simulink model "TST_InjCrv_MI1"  (R2016b)
settings: Solver=FixedStepDiscrete  StartTime=0.0  StopTime=simTime  FixedStep=sampleTime  RelTol=1e-3
values from neighbouring files (symbols this model uses):
  testCase = 1    [initTST_InjCrv_MI1_001.m]    (also in initTST_InjCrv_MI1_002.m = 2; initTST_InjCrv_MI1_003.m = 3; initTST_InjCrv_MI1_004.m = 4; initTST_InjCrv_MI1_005.m = 5)
libraries: simulink x26, UnitTest_Lib x20
settings Model: Creator=zhengjinyan  LastModifiedBy=zhengjinyan
settings DebuggingCC: SignalRangeChecking=error

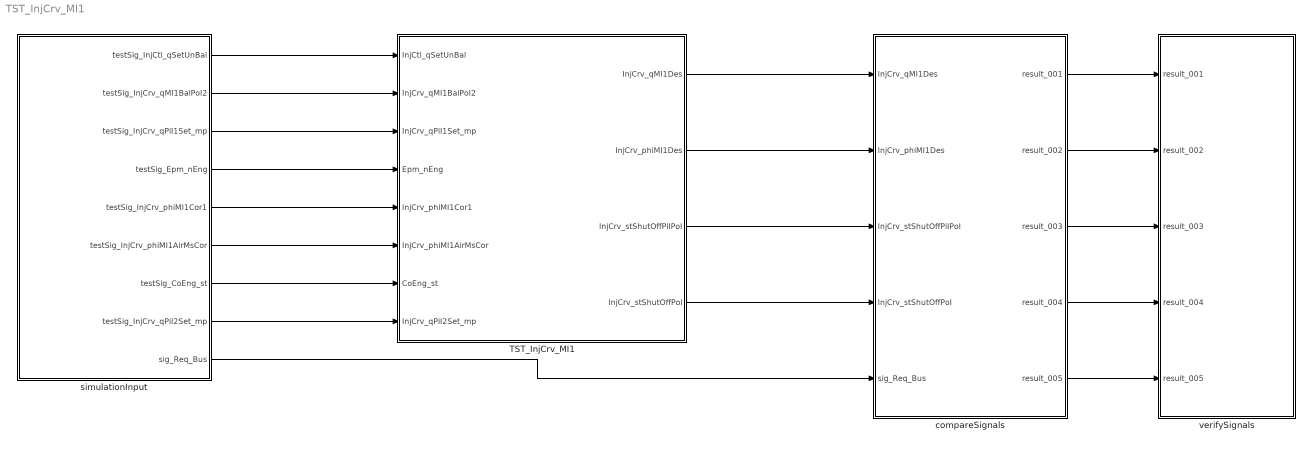
== system TST_InjCrv_MI1 ==
  TST_InjCrv_MI1 : Subsystem
  compareSignals : Subsystem
  simulationInput : Subsystem
  verifySignals : Subsystem
  wires:
  simulationInput/1(testSig_InjCtl_qSetUnBal) -> TST_InjCrv_MI1/1(InjCtl_qSetUnBal)
  simulationInput/2(testSig_InjCrv_qMI1BalPoI2) -> TST_InjCrv_MI1/2(InjCrv_qMI1BalPoI2)
  simulationInput/3(testSig_InjCrv_qPiI1Set_mp) -> TST_InjCrv_MI1/3(InjCrv_qPiI1Set_mp)
  simulationInput/4(testSig_Epm_nEng) -> TST_InjCrv_MI1/4(Epm_nEng)
  simulationInput/5(testSig_InjCrv_phiMI1Cor1) -> TST_InjCrv_MI1/5(InjCrv_phiMI1Cor1)
  simulationInput/6(testSig_InjCrv_phiMI1AirMsCor) -> TST_InjCrv_MI1/6(InjCrv_phiMI1AirMsCor)
  simulationInput/7(testSig_CoEng_st) -> TST_InjCrv_MI1/7(CoEng_st)
  simulationInput/8(testSig_InjCrv_qPiI2Set_mp) -> TST_InjCrv_MI1/8(InjCrv_qPiI2Set_mp)
  TST_InjCrv_MI1/1(InjCrv_qMI1Des) -> compareSignals/1(InjCrv_qMI1Des)
  TST_InjCrv_MI1/2(InjCrv_phiMI1Des) -> compareSignals/2(InjCrv_phiMI1Des)
  TST_InjCrv_MI1/3(InjCrv_stShutOffPiIPoI) -> compareSignals/3(InjCrv_stShutOffPiIPoI)
  TST_InjCrv_MI1/4(InjCrv_stShutOffPoI) -> compareSignals/4(InjCrv_stShutOffPoI)
  simulationInput/9(sig_Req_Bus) -> compareSignals/5(sig_Req_Bus)
  compareSignals/1(result_001) -> verifySignals/1(result_001)
  compareSignals/2(result_002) -> verifySignals/2(result_002)
  compareSignals/3(result_003) -> verifySignals/3(result_003)
  compareSignals/4(result_004) -> verifySignals/4(result_004)
  compareSignals/5(result_005) -> verifySignals/5(result_005)

== system TST_InjCrv_MI1/TST_InjCrv_MI1 ==
  InjCtl_qSetUnBal : Inport
  InjCrv_qMI1BalPoI2 : Inport  Port=2
  InjCrv_qPiI1Set_mp : Inport  Port=3
  Epm_nEng : Inport  Port=4
  InjCrv_phiMI1Cor1 : Inport  Port=5
  InjCrv_phiMI1AirMsCor : Inport  Port=6
  CoEng_st : Inport  Port=7
  InjCrv_qPiI2Set_mp : Inport  Port=8
  Function_Call : simulink/Ports & Subsystems/Function-Call Generator  sample_time=sampleTime  numberOfIterations=1
  InjCrv_MI1 : ModelReference  ModelNameDialog=InjCrv_MI1  SimulationMode=Normal  ModelReferenceVersion=1.46  TriggerPortName=function  TriggerPortTriggerType=function-call  TriggerPortStatesWhenEnabling=held
  InjCrv_qMI1Des : Outport
  InjCrv_phiMI1Des : Outport  Port=2
  InjCrv_stShutOffPiIPoI : Outport  Port=3
  InjCrv_stShutOffPoI : Outport  Port=4
  wires:
  Function_Call/1 -> InjCrv_MI1/Trigger
  InjCtl_qSetUnBal/1 -> InjCrv_MI1/1
  InjCrv_qMI1BalPoI2/1 -> InjCrv_MI1/2
  InjCrv_qPiI1Set_mp/1 -> InjCrv_MI1/3
  Epm_nEng/1 -> InjCrv_MI1/4
  InjCrv_phiMI1Cor1/1 -> InjCrv_MI1/5
  InjCrv_phiMI1AirMsCor/1 -> InjCrv_MI1/6
  CoEng_st/1 -> InjCrv_MI1/7
  InjCrv_qPiI2Set_mp/1 -> InjCrv_MI1/8
  InjCrv_MI1/1 -> InjCrv_qMI1Des/1
  InjCrv_MI1/2 -> InjCrv_phiMI1Des/1
  InjCrv_MI1/3 -> InjCrv_stShutOffPiIPoI/1
  InjCrv_MI1/4 -> InjCrv_stShutOffPoI/1

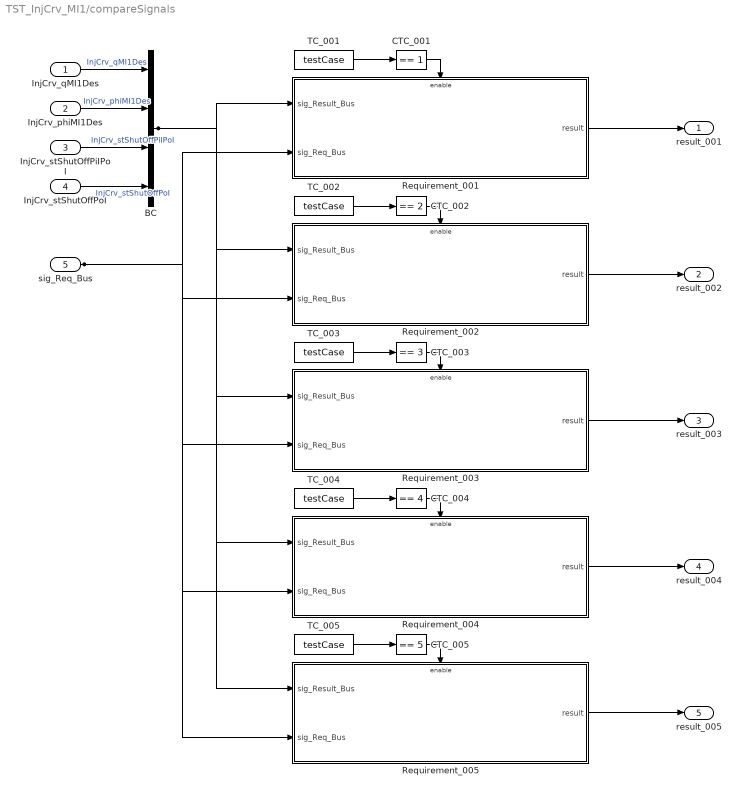
== system TST_InjCrv_MI1/compareSignals ==
  InjCrv_qMI1Des : Inport
  InjCrv_phiMI1Des : Inport  Port=2
  InjCrv_stShutOffPiIPoI : Inport  Port=3
  InjCrv_stShutOffPoI : Inport  Port=4
  sig_Req_Bus : Inport  Port=5
  BC : BusCreator  Inputs=4
  CTC_001 : simulink/Logic and Bit Operations/Compare To Constant  relop===  const=1  OutDataTypeStr=boolean
  CTC_002 : simulink/Logic and Bit Operations/Compare To Constant  relop===  const=2  OutDataTypeStr=boolean
  CTC_003 : simulink/Logic and Bit Operations/Compare To Constant  relop===  const=3  OutDataTypeStr=boolean
  CTC_004 : simulink/Logic and Bit Operations/Compare To Constant  relop===  const=4  OutDataTypeStr=boolean
  CTC_005 : simulink/Logic and Bit Operations/Compare To Constant  relop===  const=5  OutDataTypeStr=boolean
  Requirement_001 : Subsystem
  Requirement_002 : Subsystem
  Requirement_003 : Subsystem
  Requirement_004 : Subsystem
  Requirement_005 : Subsystem
  TC_001 : Constant  Value=testCase
  TC_002 : Constant  Value=testCase
  TC_003 : Constant  Value=testCase
  TC_004 : Constant  Value=testCase
  TC_005 : Constant  Value=testCase
  result_001 : Outport
  result_002 : Outport  Port=2
  result_003 : Outport  Port=3
  result_004 : Outport  Port=4
  result_005 : Outport  Port=5
  wires:
  InjCrv_qMI1Des/1 -> BC/1  "InjCrv_qMI1Des"
  InjCrv_phiMI1Des/1 -> BC/2  "InjCrv_phiMI1Des"
  InjCrv_stShutOffPiIPoI/1 -> BC/3  "InjCrv_stShutOffPiIPoI"
  InjCrv_stShutOffPoI/1 -> BC/4  "InjCrv_stShutOffPoI"
  TC_001/1 -> CTC_001/1
  CTC_001/1 -> Requirement_001/Enable
  sig_Req_Bus/1 -> Requirement_001/2(sig_Req_Bus), Requirement_002/2(sig_Req_Bus), Requirement_003/2(sig_Req_Bus), Requirement_004/2(sig_Req_Bus), Requirement_005/2(sig_Req_Bus)
  BC/1 -> Requirement_001/1(sig_Result_Bus), Requirement_002/1(sig_Result_Bus), Requirement_003/1(sig_Result_Bus), Requirement_004/1(sig_Result_Bus), Requirement_005/1(sig_Result_Bus)
  Requirement_001/1(result) -> result_001/1
  TC_002/1 -> CTC_002/1
  CTC_002/1 -> Requirement_002/Enable
  Requirement_002/1(result) -> result_002/1
  TC_003/1 -> CTC_003/1
  CTC_003/1 -> Requirement_003/Enable
  Requirement_003/1(result) -> result_003/1
  TC_004/1 -> CTC_004/1
  CTC_004/1 -> Requirement_004/Enable
  Requirement_004/1(result) -> result_004/1
  TC_005/1 -> CTC_005/1
  CTC_005/1 -> Requirement_005/Enable
  Requirement_005/1(result) -> result_005/1

== system TST_InjCrv_MI1/simulationInput ==
  BS : BusSelector  OutputSignals=testSig_InjCtl_qSetUnBal,testSig_InjCrv_qMI1BalPoI2,testSig_InjCrv_qPiI1Set_mp,testSig_Epm_nEng,testSig_InjCrv_phiMI1Cor1,testSig_InjCrv_phiMI1AirMsCor,testSig_CoEng_st,testSig_InjCrv_qPiI2Set_mp
  MPSw : MultiPortSwitch  Inputs=5  SaturateOnIntegerOverflow=on  InputSameDT=on
  TestCase : Constant  Value=testCase
  testSignals_R001 : Subsystem
  testSignals_R002 : Subsystem
  testSignals_R003 : Subsystem
  testSignals_R004 : Subsystem
  testSignals_R005 : Subsystem
  testSig_InjCtl_qSetUnBal : Outport
  testSig_InjCrv_qMI1BalPoI2 : Outport  Port=2
  testSig_InjCrv_qPiI1Set_mp : Outport  Port=3
  testSig_Epm_nEng : Outport  Port=4
  testSig_InjCrv_phiMI1Cor1 : Outport  Port=5
  testSig_InjCrv_phiMI1AirMsCor : Outport  Port=6
  testSig_CoEng_st : Outport  Port=7
  testSig_InjCrv_qPiI2Set_mp : Outport  Port=8
  sig_Req_Bus : Outport  Port=9
  wires:
  BS/1 -> testSig_InjCtl_qSetUnBal/1  "<testSig_InjCtl_qSetUnBal>"
  BS/2 -> testSig_InjCrv_qMI1BalPoI2/1  "<testSig_InjCrv_qMI1BalPoI2>"
  BS/3 -> testSig_InjCrv_qPiI1Set_mp/1  "<testSig_InjCrv_qPiI1Set_mp>"
  BS/4 -> testSig_Epm_nEng/1  "<testSig_Epm_nEng>"
  BS/5 -> testSig_InjCrv_phiMI1Cor1/1  "<testSig_InjCrv_phiMI1Cor1>"
  BS/6 -> testSig_InjCrv_phiMI1AirMsCor/1  "<testSig_InjCrv_phiMI1AirMsCor>"
  BS/7 -> testSig_CoEng_st/1  "<testSig_CoEng_st>"
  BS/8 -> testSig_InjCrv_qPiI2Set_mp/1  "<testSig_InjCrv_qPiI2Set_mp>"
  MPSw/1 -> BS/1, sig_Req_Bus/1
  TestCase/1 -> MPSw/1
  testSignals_R001/1(testSignals) -> MPSw/2
  testSignals_R002/1(testSignals) -> MPSw/3
  testSignals_R003/1(testSignals) -> MPSw/4
  testSignals_R004/1(testSignals) -> MPSw/5
  testSignals_R005/1(testSignals) -> MPSw/6

== system TST_InjCrv_MI1/verifySignals ==
  result_001 : Inport
  result_002 : Inport  Port=2
  result_003 : Inport  Port=3
  result_004 : Inport  Port=4
  result_005 : Inport  Port=5
  Assertion_001 : Assertion  Enabled=off
  Assertion_002 : Assertion  Enabled=off
  Assertion_003 : Assertion  Enabled=off
  Assertion_004 : Assertion  Enabled=off
  Assertion_005 : Assertion  Enabled=off
  wires:
  result_001/1 -> Assertion_001/1
  result_002/1 -> Assertion_002/1
  result_003/1 -> Assertion_003/1
  result_004/1 -> Assertion_004/1
  result_005/1 -> Assertion_005/1

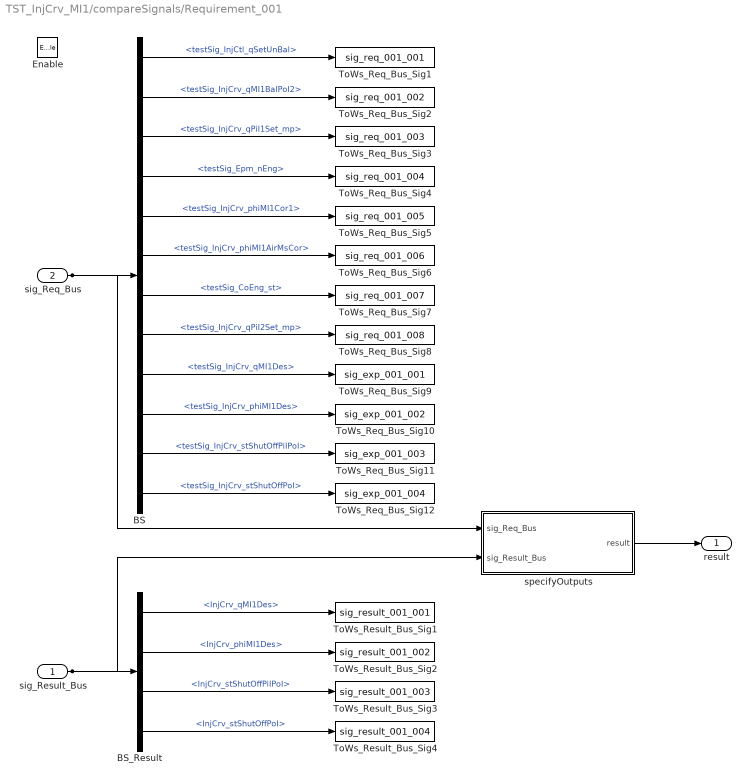
== system TST_InjCrv_MI1/compareSignals/Requirement_001 ==
  sig_Result_Bus : Inport
  sig_Req_Bus : Inport  Port=2
  Enable : EnablePort
  BS : BusSelector  OutputSignals=testSig_InjCtl_qSetUnBal,testSig_InjCrv_qMI1BalPoI2,testSig_InjCrv_qPiI1Set_mp,testSig_Epm_nEng,testSig_InjCrv_phiMI1Cor1,testSig_InjCrv_phiMI1AirMsCor,testSig_CoEng_st,testSig_InjCrv_qPiI2Set_mp,testSig_InjCrv_qMI1Des,testSig_InjCrv_phiMI1Des,testSig_InjCrv_stShutOffPiIPoI,testSig_InjCrv_stShutOffPoI
  BS_Result : BusSelector  OutputSignals=InjCrv_qMI1Des,InjCrv_phiMI1Des,InjCrv_stShutOffPiIPoI,InjCrv_stShutOffPoI
  ToWs_Req_Bus_Sig1 : ToWorkspace  VariableName=sig_req_001_001  SaveFormat=Structure With Time
  ToWs_Req_Bus_Sig10 : ToWorkspace  VariableName=sig_exp_001_002  SaveFormat=Structure With Time
  ToWs_Req_Bus_Sig11 : ToWorkspace  VariableName=sig_exp_001_003  SaveFormat=Structure With Time
  ToWs_Req_Bus_Sig12 : ToWorkspace  VariableName=sig_exp_001_004  SaveFormat=Structure With Time
  ToWs_Req_Bus_Sig2 : ToWorkspace  VariableName=sig_req_001_002  SaveFormat=Structure With Time
  ToWs_Req_Bus_Sig3 : ToWorkspace  VariableName=sig_req_001_003  SaveFormat=Structure With Time
  ToWs_Req_Bus_Sig4 : ToWorkspace  VariableName=sig_req_001_004  SaveFormat=Structure With Time
  ToWs_Req_Bus_Sig5 : ToWorkspace  VariableName=sig_req_001_005  SaveFormat=Structure With Time
  ToWs_Req_Bus_Sig6 : ToWorkspace  VariableName=sig_req_001_006  SaveFormat=Structure With Time
  ToWs_Req_Bus_Sig7 : ToWorkspace  VariableName=sig_req_001_007  SaveFormat=Structure With Time
  ToWs_Req_Bus_Sig8 : ToWorkspace  VariableName=sig_req_001_008  SaveFormat=Structure With Time
  ToWs_Req_Bus_Sig9 : ToWorkspace  VariableName=sig_exp_001_001  SaveFormat=Structure With Time
  ToWs_Result_Bus_Sig1 : ToWorkspace  VariableName=sig_result_001_001  SaveFormat=Structure With Time
  ToWs_Result_Bus_Sig2 : ToWorkspace  VariableName=sig_result_001_002  SaveFormat=Structure With Time
  ToWs_Result_Bus_Sig3 : ToWorkspace  VariableName=sig_result_001_003  SaveFormat=Structure With Time
  ToWs_Result_Bus_Sig4 : ToWorkspace  VariableName=sig_result_001_004  SaveFormat=Structure With Time
  specifyOutputs : Subsystem
  result : Outport
  wires:
  sig_Req_Bus/1 -> BS/1, specifyOutputs/1(sig_Req_Bus)
  BS/1 -> ToWs_Req_Bus_Sig1/1  "<testSig_InjCtl_qSetUnBal>"
  BS/2 -> ToWs_Req_Bus_Sig2/1  "<testSig_InjCrv_qMI1BalPoI2>"
  BS/3 -> ToWs_Req_Bus_Sig3/1  "<testSig_InjCrv_qPiI1Set_mp>"
  BS/4 -> ToWs_Req_Bus_Sig4/1  "<testSig_Epm_nEng>"
  BS/5 -> ToWs_Req_Bus_Sig5/1  "<testSig_InjCrv_phiMI1Cor1>"
  BS/6 -> ToWs_Req_Bus_Sig6/1  "<testSig_InjCrv_phiMI1AirMsCor>"
  BS/7 -> ToWs_Req_Bus_Sig7/1  "<testSig_CoEng_st>"
  BS/8 -> ToWs_Req_Bus_Sig8/1  "<testSig_InjCrv_qPiI2Set_mp>"
  BS/9 -> ToWs_Req_Bus_Sig9/1  "<testSig_InjCrv_qMI1Des>"
  BS/10 -> ToWs_Req_Bus_Sig10/1  "<testSig_InjCrv_phiMI1Des>"
  BS/11 -> ToWs_Req_Bus_Sig11/1  "<testSig_InjCrv_stShutOffPiIPoI>"
  BS/12 -> ToWs_Req_Bus_Sig12/1  "<testSig_InjCrv_stShutOffPoI>"
  sig_Result_Bus/1 -> BS_Result/1, specifyOutputs/2(sig_Result_Bus)
  BS_Result/1 -> ToWs_Result_Bus_Sig1/1  "<InjCrv_qMI1Des>"
  BS_Result/2 -> ToWs_Result_Bus_Sig2/1  "<InjCrv_phiMI1Des>"
  BS_Result/3 -> ToWs_Result_Bus_Sig3/1  "<InjCrv_stShutOffPiIPoI>"
  BS_Result/4 -> ToWs_Result_Bus_Sig4/1  "<InjCrv_stShutOffPoI>"
  specifyOutputs/1(result) -> result/1

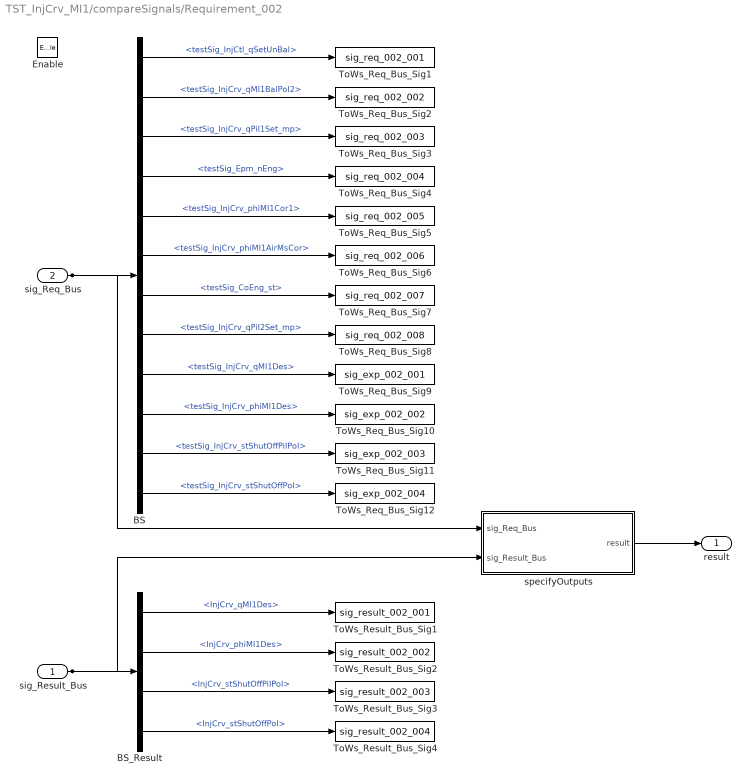
== system TST_InjCrv_MI1/compareSignals/Requirement_002 ==
  sig_Result_Bus : Inport
  sig_Req_Bus : Inport  Port=2
  Enable : EnablePort
  BS : BusSelector  OutputSignals=testSig_InjCtl_qSetUnBal,testSig_InjCrv_qMI1BalPoI2,testSig_InjCrv_qPiI1Set_mp,testSig_Epm_nEng,testSig_InjCrv_phiMI1Cor1,testSig_InjCrv_phiMI1AirMsCor,testSig_CoEng_st,testSig_InjCrv_qPiI2Set_mp,testSig_InjCrv_qMI1Des,testSig_InjCrv_phiMI1Des,testSig_InjCrv_stShutOffPiIPoI,testSig_InjCrv_stShutOffPoI
  BS_Result : BusSelector  OutputSignals=InjCrv_qMI1Des,InjCrv_phiMI1Des,InjCrv_stShutOffPiIPoI,InjCrv_stShutOffPoI
  ToWs_Req_Bus_Sig1 : ToWorkspace  VariableName=sig_req_002_001  SaveFormat=Structure With Time
  ToWs_Req_Bus_Sig10 : ToWorkspace  VariableName=sig_exp_002_002  SaveFormat=Structure With Time
  ToWs_Req_Bus_Sig11 : ToWorkspace  VariableName=sig_exp_002_003  SaveFormat=Structure With Time
  ToWs_Req_Bus_Sig12 : ToWorkspace  VariableName=sig_exp_002_004  SaveFormat=Structure With Time
  ToWs_Req_Bus_Sig2 : ToWorkspace  VariableName=sig_req_002_002  SaveFormat=Structure With Time
  ToWs_Req_Bus_Sig3 : ToWorkspace  VariableName=sig_req_002_003  SaveFormat=Structure With Time
  ToWs_Req_Bus_Sig4 : ToWorkspace  VariableName=sig_req_002_004  SaveFormat=Structure With Time
  ToWs_Req_Bus_Sig5 : ToWorkspace  VariableName=sig_req_002_005  SaveFormat=Structure With Time
  ToWs_Req_Bus_Sig6 : ToWorkspace  VariableName=sig_req_002_006  SaveFormat=Structure With Time
  ToWs_Req_Bus_Sig7 : ToWorkspace  VariableName=sig_req_002_007  SaveFormat=Structure With Time
  ToWs_Req_Bus_Sig8 : ToWorkspace  VariableName=sig_req_002_008  SaveFormat=Structure With Time
  ToWs_Req_Bus_Sig9 : ToWorkspace  VariableName=sig_exp_002_001  SaveFormat=Structure With Time
  ToWs_Result_Bus_Sig1 : ToWorkspace  VariableName=sig_result_002_001  SaveFormat=Structure With Time
  ToWs_Result_Bus_Sig2 : ToWorkspace  VariableName=sig_result_002_002  SaveFormat=Structure With Time
  ToWs_Result_Bus_Sig3 : ToWorkspace  VariableName=sig_result_002_003  SaveFormat=Structure With Time
  ToWs_Result_Bus_Sig4 : ToWorkspace  VariableName=sig_result_002_004  SaveFormat=Structure With Time
  specifyOutputs : Subsystem
  result : Outport
  wires:
  sig_Req_Bus/1 -> BS/1, specifyOutputs/1(sig_Req_Bus)
  BS/1 -> ToWs_Req_Bus_Sig1/1  "<testSig_InjCtl_qSetUnBal>"
  BS/2 -> ToWs_Req_Bus_Sig2/1  "<testSig_InjCrv_qMI1BalPoI2>"
  BS/3 -> ToWs_Req_Bus_Sig3/1  "<testSig_InjCrv_qPiI1Set_mp>"
  BS/4 -> ToWs_Req_Bus_Sig4/1  "<testSig_Epm_nEng>"
  BS/5 -> ToWs_Req_Bus_Sig5/1  "<testSig_InjCrv_phiMI1Cor1>"
  BS/6 -> ToWs_Req_Bus_Sig6/1  "<testSig_InjCrv_phiMI1AirMsCor>"
  BS/7 -> ToWs_Req_Bus_Sig7/1  "<testSig_CoEng_st>"
  BS/8 -> ToWs_Req_Bus_Sig8/1  "<testSig_InjCrv_qPiI2Set_mp>"
  BS/9 -> ToWs_Req_Bus_Sig9/1  "<testSig_InjCrv_qMI1Des>"
  BS/10 -> ToWs_Req_Bus_Sig10/1  "<testSig_InjCrv_phiMI1Des>"
  BS/11 -> ToWs_Req_Bus_Sig11/1  "<testSig_InjCrv_stShutOffPiIPoI>"
  BS/12 -> ToWs_Req_Bus_Sig12/1  "<testSig_InjCrv_stShutOffPoI>"
  sig_Result_Bus/1 -> BS_Result/1, specifyOutputs/2(sig_Result_Bus)
  BS_Result/1 -> ToWs_Result_Bus_Sig1/1  "<InjCrv_qMI1Des>"
  BS_Result/2 -> ToWs_Result_Bus_Sig2/1  "<InjCrv_phiMI1Des>"
  BS_Result/3 -> ToWs_Result_Bus_Sig3/1  "<InjCrv_stShutOffPiIPoI>"
  BS_Result/4 -> ToWs_Result_Bus_Sig4/1  "<InjCrv_stShutOffPoI>"
  specifyOutputs/1(result) -> result/1

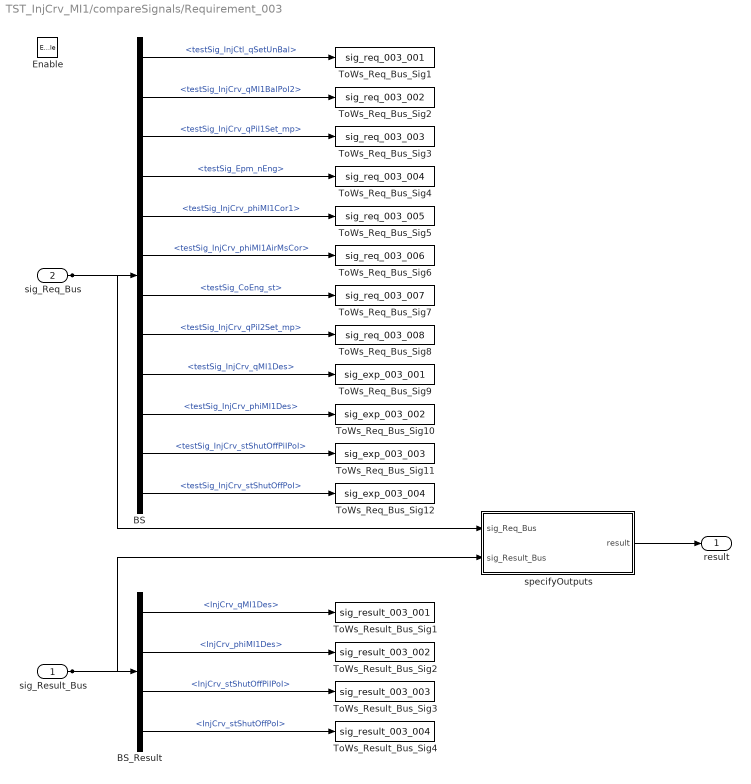
== system TST_InjCrv_MI1/compareSignals/Requirement_003 ==
  sig_Result_Bus : Inport
  sig_Req_Bus : Inport  Port=2
  Enable : EnablePort
  BS : BusSelector  OutputSignals=testSig_InjCtl_qSetUnBal,testSig_InjCrv_qMI1BalPoI2,testSig_InjCrv_qPiI1Set_mp,testSig_Epm_nEng,testSig_InjCrv_phiMI1Cor1,testSig_InjCrv_phiMI1AirMsCor,testSig_CoEng_st,testSig_InjCrv_qPiI2Set_mp,testSig_InjCrv_qMI1Des,testSig_InjCrv_phiMI1Des,testSig_InjCrv_stShutOffPiIPoI,testSig_InjCrv_stShutOffPoI
  BS_Result : BusSelector  OutputSignals=InjCrv_qMI1Des,InjCrv_phiMI1Des,InjCrv_stShutOffPiIPoI,InjCrv_stShutOffPoI
  ToWs_Req_Bus_Sig1 : ToWorkspace  VariableName=sig_req_003_001  SaveFormat=Structure With Time
  ToWs_Req_Bus_Sig10 : ToWorkspace  VariableName=sig_exp_003_002  SaveFormat=Structure With Time
  ToWs_Req_Bus_Sig11 : ToWorkspace  VariableName=sig_exp_003_003  SaveFormat=Structure With Time
  ToWs_Req_Bus_Sig12 : ToWorkspace  VariableName=sig_exp_003_004  SaveFormat=Structure With Time
  ToWs_Req_Bus_Sig2 : ToWorkspace  VariableName=sig_req_003_002  SaveFormat=Structure With Time
  ToWs_Req_Bus_Sig3 : ToWorkspace  VariableName=sig_req_003_003  SaveFormat=Structure With Time
  ToWs_Req_Bus_Sig4 : ToWorkspace  VariableName=sig_req_003_004  SaveFormat=Structure With Time
  ToWs_Req_Bus_Sig5 : ToWorkspace  VariableName=sig_req_003_005  SaveFormat=Structure With Time
  ToWs_Req_Bus_Sig6 : ToWorkspace  VariableName=sig_req_003_006  SaveFormat=Structure With Time
  ToWs_Req_Bus_Sig7 : ToWorkspace  VariableName=sig_req_003_007  SaveFormat=Structure With Time
  ToWs_Req_Bus_Sig8 : ToWorkspace  VariableName=sig_req_003_008  SaveFormat=Structure With Time
  ToWs_Req_Bus_Sig9 : ToWorkspace  VariableName=sig_exp_003_001  SaveFormat=Structure With Time
  ToWs_Result_Bus_Sig1 : ToWorkspace  VariableName=sig_result_003_001  SaveFormat=Structure With Time
  ToWs_Result_Bus_Sig2 : ToWorkspace  VariableName=sig_result_003_002  SaveFormat=Structure With Time
  ToWs_Result_Bus_Sig3 : ToWorkspace  VariableName=sig_result_003_003  SaveFormat=Structure With Time
  ToWs_Result_Bus_Sig4 : ToWorkspace  VariableName=sig_result_003_004  SaveFormat=Structure With Time
  specifyOutputs : Subsystem
  result : Outport
  wires:
  sig_Req_Bus/1 -> BS/1, specifyOutputs/1(sig_Req_Bus)
  BS/1 -> ToWs_Req_Bus_Sig1/1  "<testSig_InjCtl_qSetUnBal>"
  BS/2 -> ToWs_Req_Bus_Sig2/1  "<testSig_InjCrv_qMI1BalPoI2>"
  BS/3 -> ToWs_Req_Bus_Sig3/1  "<testSig_InjCrv_qPiI1Set_mp>"
  BS/4 -> ToWs_Req_Bus_Sig4/1  "<testSig_Epm_nEng>"
  BS/5 -> ToWs_Req_Bus_Sig5/1  "<testSig_InjCrv_phiMI1Cor1>"
  BS/6 -> ToWs_Req_Bus_Sig6/1  "<testSig_InjCrv_phiMI1AirMsCor>"
  BS/7 -> ToWs_Req_Bus_Sig7/1  "<testSig_CoEng_st>"
  BS/8 -> ToWs_Req_Bus_Sig8/1  "<testSig_InjCrv_qPiI2Set_mp>"
  BS/9 -> ToWs_Req_Bus_Sig9/1  "<testSig_InjCrv_qMI1Des>"
  BS/10 -> ToWs_Req_Bus_Sig10/1  "<testSig_InjCrv_phiMI1Des>"
  BS/11 -> ToWs_Req_Bus_Sig11/1  "<testSig_InjCrv_stShutOffPiIPoI>"
  BS/12 -> ToWs_Req_Bus_Sig12/1  "<testSig_InjCrv_stShutOffPoI>"
  sig_Result_Bus/1 -> BS_Result/1, specifyOutputs/2(sig_Result_Bus)
  BS_Result/1 -> ToWs_Result_Bus_Sig1/1  "<InjCrv_qMI1Des>"
  BS_Result/2 -> ToWs_Result_Bus_Sig2/1  "<InjCrv_phiMI1Des>"
  BS_Result/3 -> ToWs_Result_Bus_Sig3/1  "<InjCrv_stShutOffPiIPoI>"
  BS_Result/4 -> ToWs_Result_Bus_Sig4/1  "<InjCrv_stShutOffPoI>"
  specifyOutputs/1(result) -> result/1

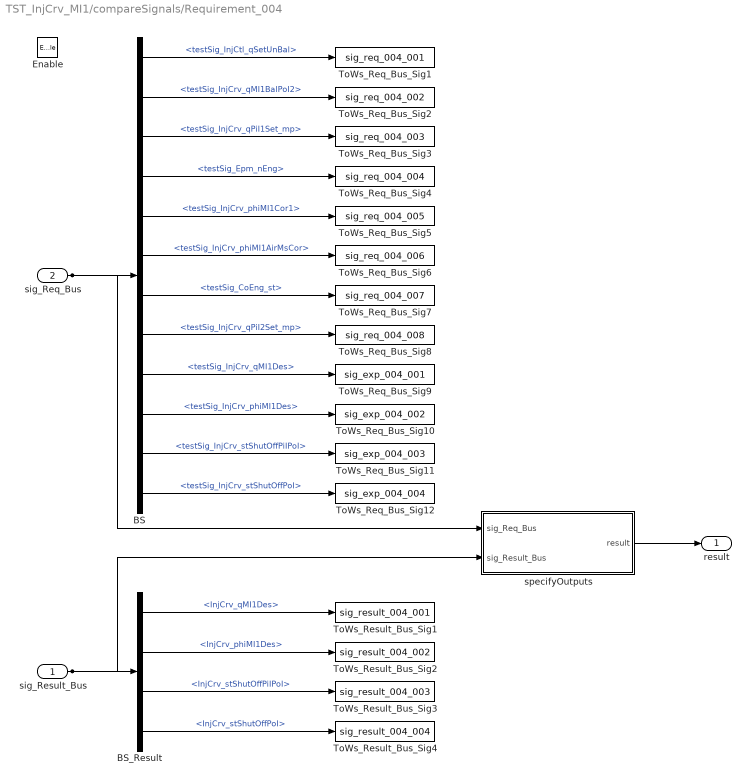
== system TST_InjCrv_MI1/compareSignals/Requirement_004 ==
  sig_Result_Bus : Inport
  sig_Req_Bus : Inport  Port=2
  Enable : EnablePort
  BS : BusSelector  OutputSignals=testSig_InjCtl_qSetUnBal,testSig_InjCrv_qMI1BalPoI2,testSig_InjCrv_qPiI1Set_mp,testSig_Epm_nEng,testSig_InjCrv_phiMI1Cor1,testSig_InjCrv_phiMI1AirMsCor,testSig_CoEng_st,testSig_InjCrv_qPiI2Set_mp,testSig_InjCrv_qMI1Des,testSig_InjCrv_phiMI1Des,testSig_InjCrv_stShutOffPiIPoI,testSig_InjCrv_stShutOffPoI
  BS_Result : BusSelector  OutputSignals=InjCrv_qMI1Des,InjCrv_phiMI1Des,InjCrv_stShutOffPiIPoI,InjCrv_stShutOffPoI
  ToWs_Req_Bus_Sig1 : ToWorkspace  VariableName=sig_req_004_001  SaveFormat=Structure With Time
  ToWs_Req_Bus_Sig10 : ToWorkspace  VariableName=sig_exp_004_002  SaveFormat=Structure With Time
  ToWs_Req_Bus_Sig11 : ToWorkspace  VariableName=sig_exp_004_003  SaveFormat=Structure With Time
  ToWs_Req_Bus_Sig12 : ToWorkspace  VariableName=sig_exp_004_004  SaveFormat=Structure With Time
  ToWs_Req_Bus_Sig2 : ToWorkspace  VariableName=sig_req_004_002  SaveFormat=Structure With Time
  ToWs_Req_Bus_Sig3 : ToWorkspace  VariableName=sig_req_004_003  SaveFormat=Structure With Time
  ToWs_Req_Bus_Sig4 : ToWorkspace  VariableName=sig_req_004_004  SaveFormat=Structure With Time
  ToWs_Req_Bus_Sig5 : ToWorkspace  VariableName=sig_req_004_005  SaveFormat=Structure With Time
  ToWs_Req_Bus_Sig6 : ToWorkspace  VariableName=sig_req_004_006  SaveFormat=Structure With Time
  ToWs_Req_Bus_Sig7 : ToWorkspace  VariableName=sig_req_004_007  SaveFormat=Structure With Time
  ToWs_Req_Bus_Sig8 : ToWorkspace  VariableName=sig_req_004_008  SaveFormat=Structure With Time
  ToWs_Req_Bus_Sig9 : ToWorkspace  VariableName=sig_exp_004_001  SaveFormat=Structure With Time
  ToWs_Result_Bus_Sig1 : ToWorkspace  VariableName=sig_result_004_001  SaveFormat=Structure With Time
  ToWs_Result_Bus_Sig2 : ToWorkspace  VariableName=sig_result_004_002  SaveFormat=Structure With Time
  ToWs_Result_Bus_Sig3 : ToWorkspace  VariableName=sig_result_004_003  SaveFormat=Structure With Time
  ToWs_Result_Bus_Sig4 : ToWorkspace  VariableName=sig_result_004_004  SaveFormat=Structure With Time
  specifyOutputs : Subsystem
  result : Outport
  wires:
  sig_Req_Bus/1 -> BS/1, specifyOutputs/1(sig_Req_Bus)
  BS/1 -> ToWs_Req_Bus_Sig1/1  "<testSig_InjCtl_qSetUnBal>"
  BS/2 -> ToWs_Req_Bus_Sig2/1  "<testSig_InjCrv_qMI1BalPoI2>"
  BS/3 -> ToWs_Req_Bus_Sig3/1  "<testSig_InjCrv_qPiI1Set_mp>"
  BS/4 -> ToWs_Req_Bus_Sig4/1  "<testSig_Epm_nEng>"
  BS/5 -> ToWs_Req_Bus_Sig5/1  "<testSig_InjCrv_phiMI1Cor1>"
  BS/6 -> ToWs_Req_Bus_Sig6/1  "<testSig_InjCrv_phiMI1AirMsCor>"
  BS/7 -> ToWs_Req_Bus_Sig7/1  "<testSig_CoEng_st>"
  BS/8 -> ToWs_Req_Bus_Sig8/1  "<testSig_InjCrv_qPiI2Set_mp>"
  BS/9 -> ToWs_Req_Bus_Sig9/1  "<testSig_InjCrv_qMI1Des>"
  BS/10 -> ToWs_Req_Bus_Sig10/1  "<testSig_InjCrv_phiMI1Des>"
  BS/11 -> ToWs_Req_Bus_Sig11/1  "<testSig_InjCrv_stShutOffPiIPoI>"
  BS/12 -> ToWs_Req_Bus_Sig12/1  "<testSig_InjCrv_stShutOffPoI>"
  sig_Result_Bus/1 -> BS_Result/1, specifyOutputs/2(sig_Result_Bus)
  BS_Result/1 -> ToWs_Result_Bus_Sig1/1  "<InjCrv_qMI1Des>"
  BS_Result/2 -> ToWs_Result_Bus_Sig2/1  "<InjCrv_phiMI1Des>"
  BS_Result/3 -> ToWs_Result_Bus_Sig3/1  "<InjCrv_stShutOffPiIPoI>"
  BS_Result/4 -> ToWs_Result_Bus_Sig4/1  "<InjCrv_stShutOffPoI>"
  specifyOutputs/1(result) -> result/1

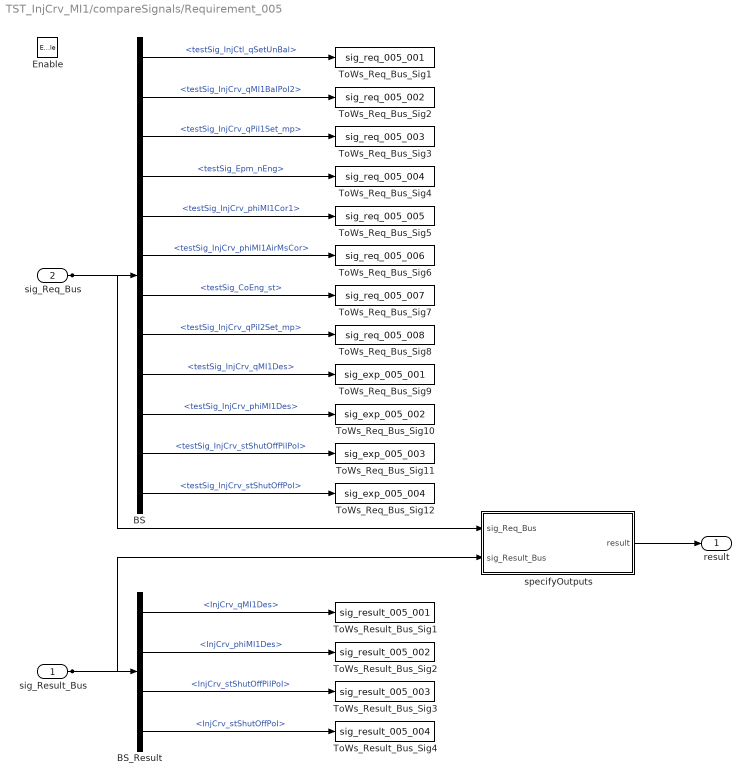
== system TST_InjCrv_MI1/compareSignals/Requirement_005 ==
  sig_Result_Bus : Inport
  sig_Req_Bus : Inport  Port=2
  Enable : EnablePort
  BS : BusSelector  OutputSignals=testSig_InjCtl_qSetUnBal,testSig_InjCrv_qMI1BalPoI2,testSig_InjCrv_qPiI1Set_mp,testSig_Epm_nEng,testSig_InjCrv_phiMI1Cor1,testSig_InjCrv_phiMI1AirMsCor,testSig_CoEng_st,testSig_InjCrv_qPiI2Set_mp,testSig_InjCrv_qMI1Des,testSig_InjCrv_phiMI1Des,testSig_InjCrv_stShutOffPiIPoI,testSig_InjCrv_stShutOffPoI
  BS_Result : BusSelector  OutputSignals=InjCrv_qMI1Des,InjCrv_phiMI1Des,InjCrv_stShutOffPiIPoI,InjCrv_stShutOffPoI
  ToWs_Req_Bus_Sig1 : ToWorkspace  VariableName=sig_req_005_001  SaveFormat=Structure With Time
  ToWs_Req_Bus_Sig10 : ToWorkspace  VariableName=sig_exp_005_002  SaveFormat=Structure With Time
  ToWs_Req_Bus_Sig11 : ToWorkspace  VariableName=sig_exp_005_003  SaveFormat=Structure With Time
  ToWs_Req_Bus_Sig12 : ToWorkspace  VariableName=sig_exp_005_004  SaveFormat=Structure With Time
  ToWs_Req_Bus_Sig2 : ToWorkspace  VariableName=sig_req_005_002  SaveFormat=Structure With Time
  ToWs_Req_Bus_Sig3 : ToWorkspace  VariableName=sig_req_005_003  SaveFormat=Structure With Time
  ToWs_Req_Bus_Sig4 : ToWorkspace  VariableName=sig_req_005_004  SaveFormat=Structure With Time
  ToWs_Req_Bus_Sig5 : ToWorkspace  VariableName=sig_req_005_005  SaveFormat=Structure With Time
  ToWs_Req_Bus_Sig6 : ToWorkspace  VariableName=sig_req_005_006  SaveFormat=Structure With Time
  ToWs_Req_Bus_Sig7 : ToWorkspace  VariableName=sig_req_005_007  SaveFormat=Structure With Time
  ToWs_Req_Bus_Sig8 : ToWorkspace  VariableName=sig_req_005_008  SaveFormat=Structure With Time
  ToWs_Req_Bus_Sig9 : ToWorkspace  VariableName=sig_exp_005_001  SaveFormat=Structure With Time
  ToWs_Result_Bus_Sig1 : ToWorkspace  VariableName=sig_result_005_001  SaveFormat=Structure With Time
  ToWs_Result_Bus_Sig2 : ToWorkspace  VariableName=sig_result_005_002  SaveFormat=Structure With Time
  ToWs_Result_Bus_Sig3 : ToWorkspace  VariableName=sig_result_005_003  SaveFormat=Structure With Time
  ToWs_Result_Bus_Sig4 : ToWorkspace  VariableName=sig_result_005_004  SaveFormat=Structure With Time
  specifyOutputs : Subsystem
  result : Outport
  wires:
  sig_Req_Bus/1 -> BS/1, specifyOutputs/1(sig_Req_Bus)
  BS/1 -> ToWs_Req_Bus_Sig1/1  "<testSig_InjCtl_qSetUnBal>"
  BS/2 -> ToWs_Req_Bus_Sig2/1  "<testSig_InjCrv_qMI1BalPoI2>"
  BS/3 -> ToWs_Req_Bus_Sig3/1  "<testSig_InjCrv_qPiI1Set_mp>"
  BS/4 -> ToWs_Req_Bus_Sig4/1  "<testSig_Epm_nEng>"
  BS/5 -> ToWs_Req_Bus_Sig5/1  "<testSig_InjCrv_phiMI1Cor1>"
  BS/6 -> ToWs_Req_Bus_Sig6/1  "<testSig_InjCrv_phiMI1AirMsCor>"
  BS/7 -> ToWs_Req_Bus_Sig7/1  "<testSig_CoEng_st>"
  BS/8 -> ToWs_Req_Bus_Sig8/1  "<testSig_InjCrv_qPiI2Set_mp>"
  BS/9 -> ToWs_Req_Bus_Sig9/1  "<testSig_InjCrv_qMI1Des>"
  BS/10 -> ToWs_Req_Bus_Sig10/1  "<testSig_InjCrv_phiMI1Des>"
  BS/11 -> ToWs_Req_Bus_Sig11/1  "<testSig_InjCrv_stShutOffPiIPoI>"
  BS/12 -> ToWs_Req_Bus_Sig12/1  "<testSig_InjCrv_stShutOffPoI>"
  sig_Result_Bus/1 -> BS_Result/1, specifyOutputs/2(sig_Result_Bus)
  BS_Result/1 -> ToWs_Result_Bus_Sig1/1  "<InjCrv_qMI1Des>"
  BS_Result/2 -> ToWs_Result_Bus_Sig2/1  "<InjCrv_phiMI1Des>"
  BS_Result/3 -> ToWs_Result_Bus_Sig3/1  "<InjCrv_stShutOffPiIPoI>"
  BS_Result/4 -> ToWs_Result_Bus_Sig4/1  "<InjCrv_stShutOffPoI>"
  specifyOutputs/1(result) -> result/1

== system TST_InjCrv_MI1/simulationInput/testSignals_R001 ==
  BC : BusCreator  Inputs=12
  spec_CoEng_st : FromWorkspace  VariableName=testSig_CoEng_st  Interpolate=off  OutputAfterFinalValue=Holding final value
  spec_Epm_nEng : FromWorkspace  VariableName=testSig_Epm_nEng  Interpolate=off  OutputAfterFinalValue=Holding final value
  spec_InjCrv_phiMI1AirMsCor : FromWorkspace  VariableName=testSig_InjCrv_phiMI1AirMsCor  Interpolate=off  OutputAfterFinalValue=Holding final value
  spec_InjCrv_phiMI1Cor1 : FromWorkspace  VariableName=testSig_InjCrv_phiMI1Cor1  Interpolate=off  OutputAfterFinalValue=Holding final value
  spec_InjCrv_phiMI1Des : FromWorkspace  VariableName=testSig_InjCrv_phiMI1Des  Interpolate=off  OutputAfterFinalValue=Holding final value
  spec_InjCrv_qMI1BalPoI2 : FromWorkspace  VariableName=testSig_InjCrv_qMI1BalPoI2  Interpolate=off  OutputAfterFinalValue=Holding final value
  spec_InjCrv_qMI1Des : FromWorkspace  VariableName=testSig_InjCrv_qMI1Des  Interpolate=off  OutputAfterFinalValue=Holding final value
  spec_InjCrv_qPiI1Set_mp : FromWorkspace  VariableName=testSig_InjCrv_qPiI1Set_mp  Interpolate=off  OutputAfterFinalValue=Holding final value
  spec_InjCrv_qPiI2Set_mp : FromWorkspace  VariableName=testSig_InjCrv_qPiI2Set_mp  Interpolate=off  OutputAfterFinalValue=Holding final value
  spec_InjCrv_stShutOffPiIPoI : FromWorkspace  VariableName=testSig_InjCrv_stShutOffPiIPoI  Interpolate=off  OutputAfterFinalValue=Holding final value
  spec_InjCrv_stShutOffPoI : FromWorkspace  VariableName=testSig_InjCrv_stShutOffPoI  Interpolate=off  OutputAfterFinalValue=Holding final value
  spec_InjCtl_qSetUnBal : FromWorkspace  VariableName=testSig_InjCtl_qSetUnBal  Interpolate=off  OutputAfterFinalValue=Holding final value
  testSignals : Outport
  wires:
  BC/1 -> testSignals/1
  spec_InjCtl_qSetUnBal/1 -> BC/1  "testSig_InjCtl_qSetUnBal"
  spec_InjCrv_qMI1BalPoI2/1 -> BC/2  "testSig_InjCrv_qMI1BalPoI2"
  spec_InjCrv_qPiI1Set_mp/1 -> BC/3  "testSig_InjCrv_qPiI1Set_mp"
  spec_Epm_nEng/1 -> BC/4  "testSig_Epm_nEng"
  spec_InjCrv_phiMI1Cor1/1 -> BC/5  "testSig_InjCrv_phiMI1Cor1"
  spec_InjCrv_phiMI1AirMsCor/1 -> BC/6  "testSig_InjCrv_phiMI1AirMsCor"
  spec_CoEng_st/1 -> BC/7  "testSig_CoEng_st"
  spec_InjCrv_qPiI2Set_mp/1 -> BC/8  "testSig_InjCrv_qPiI2Set_mp"
  spec_InjCrv_qMI1Des/1 -> BC/9  "testSig_InjCrv_qMI1Des"
  spec_InjCrv_phiMI1Des/1 -> BC/10  "testSig_InjCrv_phiMI1Des"
  spec_InjCrv_stShutOffPiIPoI/1 -> BC/11  "testSig_InjCrv_stShutOffPiIPoI"
  spec_InjCrv_stShutOffPoI/1 -> BC/12  "testSig_InjCrv_stShutOffPoI"

== system TST_InjCrv_MI1/simulationInput/testSignals_R002 ==
  BC : BusCreator  Inputs=12
  spec_CoEng_st : FromWorkspace  VariableName=testSig_CoEng_st  Interpolate=off  OutputAfterFinalValue=Holding final value
  spec_Epm_nEng : FromWorkspace  VariableName=testSig_Epm_nEng  Interpolate=off  OutputAfterFinalValue=Holding final value
  spec_InjCrv_phiMI1AirMsCor : FromWorkspace  VariableName=testSig_InjCrv_phiMI1AirMsCor  Interpolate=off  OutputAfterFinalValue=Holding final value
  spec_InjCrv_phiMI1Cor1 : FromWorkspace  VariableName=testSig_InjCrv_phiMI1Cor1  Interpolate=off  OutputAfterFinalValue=Holding final value
  spec_InjCrv_phiMI1Des : FromWorkspace  VariableName=testSig_InjCrv_phiMI1Des  Interpolate=off  OutputAfterFinalValue=Holding final value
  spec_InjCrv_qMI1BalPoI2 : FromWorkspace  VariableName=testSig_InjCrv_qMI1BalPoI2  Interpolate=off  OutputAfterFinalValue=Holding final value
  spec_InjCrv_qMI1Des : FromWorkspace  VariableName=testSig_InjCrv_qMI1Des  Interpolate=off  OutputAfterFinalValue=Holding final value
  spec_InjCrv_qPiI1Set_mp : FromWorkspace  VariableName=testSig_InjCrv_qPiI1Set_mp  Interpolate=off  OutputAfterFinalValue=Holding final value
  spec_InjCrv_qPiI2Set_mp : FromWorkspace  VariableName=testSig_InjCrv_qPiI2Set_mp  Interpolate=off  OutputAfterFinalValue=Holding final value
  spec_InjCrv_stShutOffPiIPoI : FromWorkspace  VariableName=testSig_InjCrv_stShutOffPiIPoI  Interpolate=off  OutputAfterFinalValue=Holding final value
  spec_InjCrv_stShutOffPoI : FromWorkspace  VariableName=testSig_InjCrv_stShutOffPoI  Interpolate=off  OutputAfterFinalValue=Holding final value
  spec_InjCtl_qSetUnBal : FromWorkspace  VariableName=testSig_InjCtl_qSetUnBal  Interpolate=off  OutputAfterFinalValue=Holding final value
  testSignals : Outport
  wires:
  BC/1 -> testSignals/1
  spec_InjCtl_qSetUnBal/1 -> BC/1  "testSig_InjCtl_qSetUnBal"
  spec_InjCrv_qMI1BalPoI2/1 -> BC/2  "testSig_InjCrv_qMI1BalPoI2"
  spec_InjCrv_qPiI1Set_mp/1 -> BC/3  "testSig_InjCrv_qPiI1Set_mp"
  spec_Epm_nEng/1 -> BC/4  "testSig_Epm_nEng"
  spec_InjCrv_phiMI1Cor1/1 -> BC/5  "testSig_InjCrv_phiMI1Cor1"
  spec_InjCrv_phiMI1AirMsCor/1 -> BC/6  "testSig_InjCrv_phiMI1AirMsCor"
  spec_CoEng_st/1 -> BC/7  "testSig_CoEng_st"
  spec_InjCrv_qPiI2Set_mp/1 -> BC/8  "testSig_InjCrv_qPiI2Set_mp"
  spec_InjCrv_qMI1Des/1 -> BC/9  "testSig_InjCrv_qMI1Des"
  spec_InjCrv_phiMI1Des/1 -> BC/10  "testSig_InjCrv_phiMI1Des"
  spec_InjCrv_stShutOffPiIPoI/1 -> BC/11  "testSig_InjCrv_stShutOffPiIPoI"
  spec_InjCrv_stShutOffPoI/1 -> BC/12  "testSig_InjCrv_stShutOffPoI"

== system TST_InjCrv_MI1/simulationInput/testSignals_R003 ==
  BC : BusCreator  Inputs=12
  spec_CoEng_st : FromWorkspace  VariableName=testSig_CoEng_st  Interpolate=off  OutputAfterFinalValue=Holding final value
  spec_Epm_nEng : FromWorkspace  VariableName=testSig_Epm_nEng  Interpolate=off  OutputAfterFinalValue=Holding final value
  spec_InjCrv_phiMI1AirMsCor : FromWorkspace  VariableName=testSig_InjCrv_phiMI1AirMsCor  Interpolate=off  OutputAfterFinalValue=Holding final value
  spec_InjCrv_phiMI1Cor1 : FromWorkspace  VariableName=testSig_InjCrv_phiMI1Cor1  Interpolate=off  OutputAfterFinalValue=Holding final value
  spec_InjCrv_phiMI1Des : FromWorkspace  VariableName=testSig_InjCrv_phiMI1Des  Interpolate=off  OutputAfterFinalValue=Holding final value
  spec_InjCrv_qMI1BalPoI2 : FromWorkspace  VariableName=testSig_InjCrv_qMI1BalPoI2  Interpolate=off  OutputAfterFinalValue=Holding final value
  spec_InjCrv_qMI1Des : FromWorkspace  VariableName=testSig_InjCrv_qMI1Des  Interpolate=off  OutputAfterFinalValue=Holding final value
  spec_InjCrv_qPiI1Set_mp : FromWorkspace  VariableName=testSig_InjCrv_qPiI1Set_mp  Interpolate=off  OutputAfterFinalValue=Holding final value
  spec_InjCrv_qPiI2Set_mp : FromWorkspace  VariableName=testSig_InjCrv_qPiI2Set_mp  Interpolate=off  OutputAfterFinalValue=Holding final value
  spec_InjCrv_stShutOffPiIPoI : FromWorkspace  VariableName=testSig_InjCrv_stShutOffPiIPoI  Interpolate=off  OutputAfterFinalValue=Holding final value
  spec_InjCrv_stShutOffPoI : FromWorkspace  VariableName=testSig_InjCrv_stShutOffPoI  Interpolate=off  OutputAfterFinalValue=Holding final value
  spec_InjCtl_qSetUnBal : FromWorkspace  VariableName=testSig_InjCtl_qSetUnBal  Interpolate=off  OutputAfterFinalValue=Holding final value
  testSignals : Outport
  wires:
  BC/1 -> testSignals/1
  spec_InjCtl_qSetUnBal/1 -> BC/1  "testSig_InjCtl_qSetUnBal"
  spec_InjCrv_qMI1BalPoI2/1 -> BC/2  "testSig_InjCrv_qMI1BalPoI2"
  spec_InjCrv_qPiI1Set_mp/1 -> BC/3  "testSig_InjCrv_qPiI1Set_mp"
  spec_Epm_nEng/1 -> BC/4  "testSig_Epm_nEng"
  spec_InjCrv_phiMI1Cor1/1 -> BC/5  "testSig_InjCrv_phiMI1Cor1"
  spec_InjCrv_phiMI1AirMsCor/1 -> BC/6  "testSig_InjCrv_phiMI1AirMsCor"
  spec_CoEng_st/1 -> BC/7  "testSig_CoEng_st"
  spec_InjCrv_qPiI2Set_mp/1 -> BC/8  "testSig_InjCrv_qPiI2Set_mp"
  spec_InjCrv_qMI1Des/1 -> BC/9  "testSig_InjCrv_qMI1Des"
  spec_InjCrv_phiMI1Des/1 -> BC/10  "testSig_InjCrv_phiMI1Des"
  spec_InjCrv_stShutOffPiIPoI/1 -> BC/11  "testSig_InjCrv_stShutOffPiIPoI"
  spec_InjCrv_stShutOffPoI/1 -> BC/12  "testSig_InjCrv_stShutOffPoI"

== system TST_InjCrv_MI1/simulationInput/testSignals_R004 ==
  BC : BusCreator  Inputs=12
  spec_CoEng_st : FromWorkspace  VariableName=testSig_CoEng_st  Interpolate=off  OutputAfterFinalValue=Holding final value
  spec_Epm_nEng : FromWorkspace  VariableName=testSig_Epm_nEng  Interpolate=off  OutputAfterFinalValue=Holding final value
  spec_InjCrv_phiMI1AirMsCor : FromWorkspace  VariableName=testSig_InjCrv_phiMI1AirMsCor  Interpolate=off  OutputAfterFinalValue=Holding final value
  spec_InjCrv_phiMI1Cor1 : FromWorkspace  VariableName=testSig_InjCrv_phiMI1Cor1  Interpolate=off  OutputAfterFinalValue=Holding final value
  spec_InjCrv_phiMI1Des : FromWorkspace  VariableName=testSig_InjCrv_phiMI1Des  Interpolate=off  OutputAfterFinalValue=Holding final value
  spec_InjCrv_qMI1BalPoI2 : FromWorkspace  VariableName=testSig_InjCrv_qMI1BalPoI2  Interpolate=off  OutputAfterFinalValue=Holding final value
  spec_InjCrv_qMI1Des : FromWorkspace  VariableName=testSig_InjCrv_qMI1Des  Interpolate=off  OutputAfterFinalValue=Holding final value
  spec_InjCrv_qPiI1Set_mp : FromWorkspace  VariableName=testSig_InjCrv_qPiI1Set_mp  Interpolate=off  OutputAfterFinalValue=Holding final value
  spec_InjCrv_qPiI2Set_mp : FromWorkspace  VariableName=testSig_InjCrv_qPiI2Set_mp  Interpolate=off  OutputAfterFinalValue=Holding final value
  spec_InjCrv_stShutOffPiIPoI : FromWorkspace  VariableName=testSig_InjCrv_stShutOffPiIPoI  Interpolate=off  OutputAfterFinalValue=Holding final value
  spec_InjCrv_stShutOffPoI : FromWorkspace  VariableName=testSig_InjCrv_stShutOffPoI  Interpolate=off  OutputAfterFinalValue=Holding final value
  spec_InjCtl_qSetUnBal : FromWorkspace  VariableName=testSig_InjCtl_qSetUnBal  Interpolate=off  OutputAfterFinalValue=Holding final value
  testSignals : Outport
  wires:
  BC/1 -> testSignals/1
  spec_InjCtl_qSetUnBal/1 -> BC/1  "testSig_InjCtl_qSetUnBal"
  spec_InjCrv_qMI1BalPoI2/1 -> BC/2  "testSig_InjCrv_qMI1BalPoI2"
  spec_InjCrv_qPiI1Set_mp/1 -> BC/3  "testSig_InjCrv_qPiI1Set_mp"
  spec_Epm_nEng/1 -> BC/4  "testSig_Epm_nEng"
  spec_InjCrv_phiMI1Cor1/1 -> BC/5  "testSig_InjCrv_phiMI1Cor1"
  spec_InjCrv_phiMI1AirMsCor/1 -> BC/6  "testSig_InjCrv_phiMI1AirMsCor"
  spec_CoEng_st/1 -> BC/7  "testSig_CoEng_st"
  spec_InjCrv_qPiI2Set_mp/1 -> BC/8  "testSig_InjCrv_qPiI2Set_mp"
  spec_InjCrv_qMI1Des/1 -> BC/9  "testSig_InjCrv_qMI1Des"
  spec_InjCrv_phiMI1Des/1 -> BC/10  "testSig_InjCrv_phiMI1Des"
  spec_InjCrv_stShutOffPiIPoI/1 -> BC/11  "testSig_InjCrv_stShutOffPiIPoI"
  spec_InjCrv_stShutOffPoI/1 -> BC/12  "testSig_InjCrv_stShutOffPoI"

== system TST_InjCrv_MI1/simulationInput/testSignals_R005 ==
  BC : BusCreator  Inputs=12
  spec_CoEng_st : FromWorkspace  VariableName=testSig_CoEng_st  Interpolate=off  OutputAfterFinalValue=Holding final value
  spec_Epm_nEng : FromWorkspace  VariableName=testSig_Epm_nEng  Interpolate=off  OutputAfterFinalValue=Holding final value
  spec_InjCrv_phiMI1AirMsCor : FromWorkspace  VariableName=testSig_InjCrv_phiMI1AirMsCor  Interpolate=off  OutputAfterFinalValue=Holding final value
  spec_InjCrv_phiMI1Cor1 : FromWorkspace  VariableName=testSig_InjCrv_phiMI1Cor1  Interpolate=off  OutputAfterFinalValue=Holding final value
  spec_InjCrv_phiMI1Des : FromWorkspace  VariableName=testSig_InjCrv_phiMI1Des  Interpolate=off  OutputAfterFinalValue=Holding final value
  spec_InjCrv_qMI1BalPoI2 : FromWorkspace  VariableName=testSig_InjCrv_qMI1BalPoI2  Interpolate=off  OutputAfterFinalValue=Holding final value
  spec_InjCrv_qMI1Des : FromWorkspace  VariableName=testSig_InjCrv_qMI1Des  Interpolate=off  OutputAfterFinalValue=Holding final value
  spec_InjCrv_qPiI1Set_mp : FromWorkspace  VariableName=testSig_InjCrv_qPiI1Set_mp  Interpolate=off  OutputAfterFinalValue=Holding final value
  spec_InjCrv_qPiI2Set_mp : FromWorkspace  VariableName=testSig_InjCrv_qPiI2Set_mp  Interpolate=off  OutputAfterFinalValue=Holding final value
  spec_InjCrv_stShutOffPiIPoI : FromWorkspace  VariableName=testSig_InjCrv_stShutOffPiIPoI  Interpolate=off  OutputAfterFinalValue=Holding final value
  spec_InjCrv_stShutOffPoI : FromWorkspace  VariableName=testSig_InjCrv_stShutOffPoI  Interpolate=off  OutputAfterFinalValue=Holding final value
  spec_InjCtl_qSetUnBal : FromWorkspace  VariableName=testSig_InjCtl_qSetUnBal  Interpolate=off  OutputAfterFinalValue=Holding final value
  testSignals : Outport
  wires:
  BC/1 -> testSignals/1
  spec_InjCtl_qSetUnBal/1 -> BC/1  "testSig_InjCtl_qSetUnBal"
  spec_InjCrv_qMI1BalPoI2/1 -> BC/2  "testSig_InjCrv_qMI1BalPoI2"
  spec_InjCrv_qPiI1Set_mp/1 -> BC/3  "testSig_InjCrv_qPiI1Set_mp"
  spec_Epm_nEng/1 -> BC/4  "testSig_Epm_nEng"
  spec_InjCrv_phiMI1Cor1/1 -> BC/5  "testSig_InjCrv_phiMI1Cor1"
  spec_InjCrv_phiMI1AirMsCor/1 -> BC/6  "testSig_InjCrv_phiMI1AirMsCor"
  spec_CoEng_st/1 -> BC/7  "testSig_CoEng_st"
  spec_InjCrv_qPiI2Set_mp/1 -> BC/8  "testSig_InjCrv_qPiI2Set_mp"
  spec_InjCrv_qMI1Des/1 -> BC/9  "testSig_InjCrv_qMI1Des"
  spec_InjCrv_phiMI1Des/1 -> BC/10  "testSig_InjCrv_phiMI1Des"
  spec_InjCrv_stShutOffPiIPoI/1 -> BC/11  "testSig_InjCrv_stShutOffPiIPoI"
  spec_InjCrv_stShutOffPoI/1 -> BC/12  "testSig_InjCrv_stShutOffPoI"

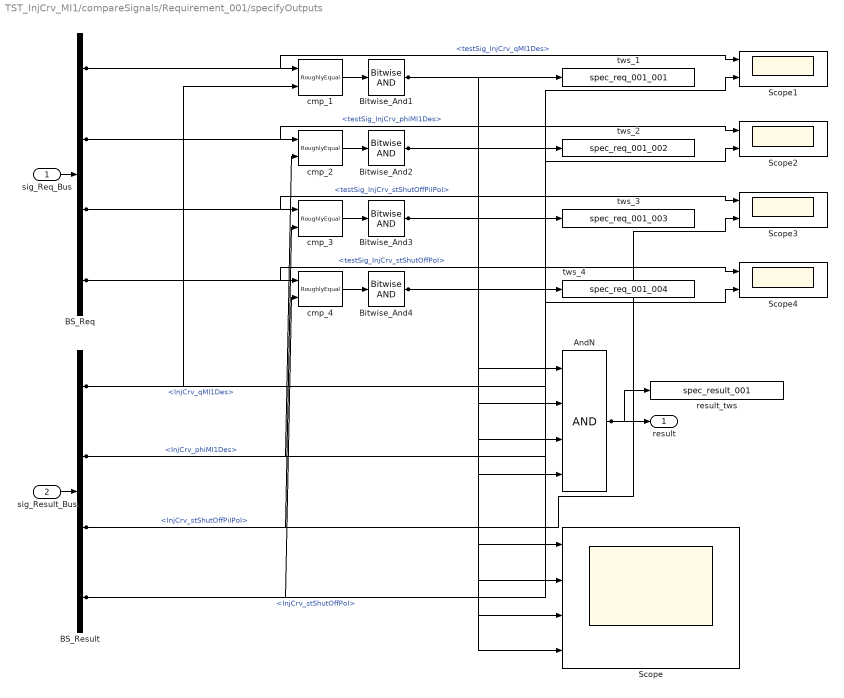
== system TST_InjCrv_MI1/compareSignals/Requirement_001/specifyOutputs ==
  sig_Req_Bus : Inport
  sig_Result_Bus : Inport  Port=2
  AndN : Logic  Inputs=4
  BS_Req : BusSelector  OutputSignals=testSig_InjCrv_qMI1Des,testSig_InjCrv_phiMI1Des,testSig_InjCrv_stShutOffPiIPoI,testSig_InjCrv_stShutOffPoI
  BS_Result : BusSelector  OutputSignals=InjCrv_qMI1Des,InjCrv_phiMI1Des,InjCrv_stShutOffPiIPoI,InjCrv_stShutOffPoI
  Bitwise_And{1..4} (4 alike) : simulink/Logic and Bit Operations/Bitwise Operator  logicop=AND  UseBitMask=off  BitMask=bin2dec('11011001')  BitMaskRealWorld=Stored Integer
  Scope : Scope  NumInputPorts=4
  Scope{1..4} (4 alike) : Scope  NumInputPorts=2
  cmp_{1..4} (4 alike) : UnitTest_Lib/RoughlyEqual  slope=0.1
  result_tws : ToWorkspace  VariableName=spec_result_001
  tws_1 : ToWorkspace  VariableName=spec_req_001_001
  tws_2 : ToWorkspace  VariableName=spec_req_001_002
  tws_3 : ToWorkspace  VariableName=spec_req_001_003
  tws_4 : ToWorkspace  VariableName=spec_req_001_004
  result : Outport
  wires:
  sig_Req_Bus/1 -> BS_Req/1
  sig_Result_Bus/1 -> BS_Result/1
  AndN/1 -> result/1, result_tws/1
  BS_Req/1 -> cmp_1/1, Scope1/1  "<testSig_InjCrv_qMI1Des>"
  BS_Result/1 -> cmp_1/2, Scope1/2  "<InjCrv_qMI1Des>"
  cmp_1/1 -> Bitwise_And1/1
  Bitwise_And1/1 -> tws_1/1, AndN/1, Scope/1
  BS_Req/2 -> cmp_2/1, Scope2/1  "<testSig_InjCrv_phiMI1Des>"
  BS_Result/2 -> cmp_2/2, Scope2/2  "<InjCrv_phiMI1Des>"
  cmp_2/1 -> Bitwise_And2/1
  Bitwise_And2/1 -> tws_2/1, AndN/2, Scope/2
  BS_Req/3 -> cmp_3/1, Scope3/1  "<testSig_InjCrv_stShutOffPiIPoI>"
  BS_Result/3 -> cmp_3/2, Scope3/2  "<InjCrv_stShutOffPiIPoI>"
  cmp_3/1 -> Bitwise_And3/1
  Bitwise_And3/1 -> tws_3/1, AndN/3, Scope/3
  BS_Req/4 -> cmp_4/1, Scope4/1  "<testSig_InjCrv_stShutOffPoI>"
  BS_Result/4 -> cmp_4/2, Scope4/2  "<InjCrv_stShutOffPoI>"
  cmp_4/1 -> Bitwise_And4/1
  Bitwise_And4/1 -> tws_4/1, AndN/4, Scope/4

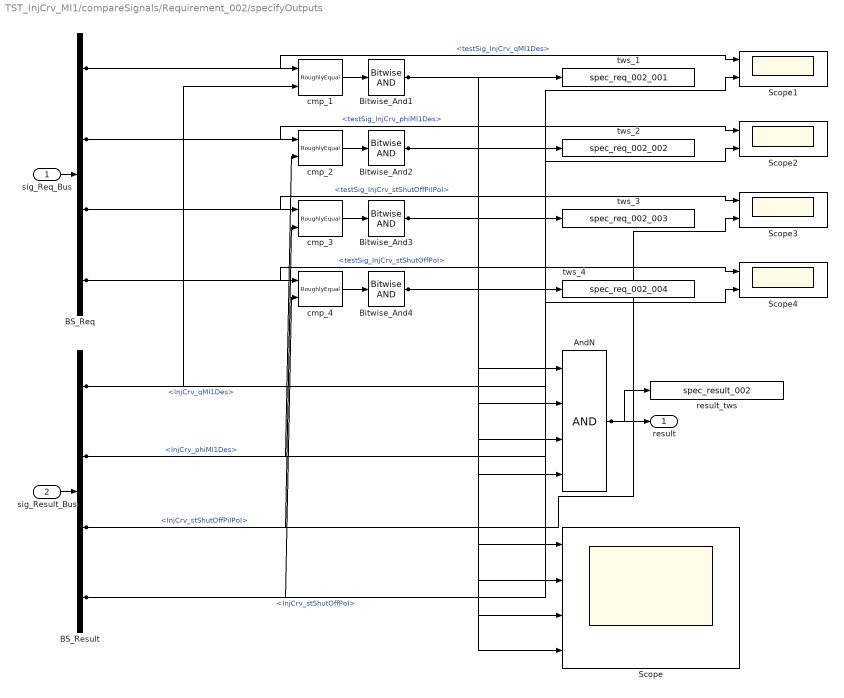
== system TST_InjCrv_MI1/compareSignals/Requirement_002/specifyOutputs ==
  sig_Req_Bus : Inport
  sig_Result_Bus : Inport  Port=2
  AndN : Logic  Inputs=4
  BS_Req : BusSelector  OutputSignals=testSig_InjCrv_qMI1Des,testSig_InjCrv_phiMI1Des,testSig_InjCrv_stShutOffPiIPoI,testSig_InjCrv_stShutOffPoI
  BS_Result : BusSelector  OutputSignals=InjCrv_qMI1Des,InjCrv_phiMI1Des,InjCrv_stShutOffPiIPoI,InjCrv_stShutOffPoI
  Bitwise_And{1..4} (4 alike) : simulink/Logic and Bit Operations/Bitwise Operator  logicop=AND  UseBitMask=off  BitMask=bin2dec('11011001')  BitMaskRealWorld=Stored Integer
  Scope : Scope  NumInputPorts=4
  Scope{1..4} (4 alike) : Scope  NumInputPorts=2
  cmp_{1..4} (4 alike) : UnitTest_Lib/RoughlyEqual  slope=0.1
  result_tws : ToWorkspace  VariableName=spec_result_002
  tws_1 : ToWorkspace  VariableName=spec_req_002_001
  tws_2 : ToWorkspace  VariableName=spec_req_002_002
  tws_3 : ToWorkspace  VariableName=spec_req_002_003
  tws_4 : ToWorkspace  VariableName=spec_req_002_004
  result : Outport
  wires:
  sig_Req_Bus/1 -> BS_Req/1
  sig_Result_Bus/1 -> BS_Result/1
  AndN/1 -> result/1, result_tws/1
  BS_Req/1 -> cmp_1/1, Scope1/1  "<testSig_InjCrv_qMI1Des>"
  BS_Result/1 -> cmp_1/2, Scope1/2  "<InjCrv_qMI1Des>"
  cmp_1/1 -> Bitwise_And1/1
  Bitwise_And1/1 -> tws_1/1, AndN/1, Scope/1
  BS_Req/2 -> cmp_2/1, Scope2/1  "<testSig_InjCrv_phiMI1Des>"
  BS_Result/2 -> cmp_2/2, Scope2/2  "<InjCrv_phiMI1Des>"
  cmp_2/1 -> Bitwise_And2/1
  Bitwise_And2/1 -> tws_2/1, AndN/2, Scope/2
  BS_Req/3 -> cmp_3/1, Scope3/1  "<testSig_InjCrv_stShutOffPiIPoI>"
  BS_Result/3 -> cmp_3/2, Scope3/2  "<InjCrv_stShutOffPiIPoI>"
  cmp_3/1 -> Bitwise_And3/1
  Bitwise_And3/1 -> tws_3/1, AndN/3, Scope/3
  BS_Req/4 -> cmp_4/1, Scope4/1  "<testSig_InjCrv_stShutOffPoI>"
  BS_Result/4 -> cmp_4/2, Scope4/2  "<InjCrv_stShutOffPoI>"
  cmp_4/1 -> Bitwise_And4/1
  Bitwise_And4/1 -> tws_4/1, AndN/4, Scope/4

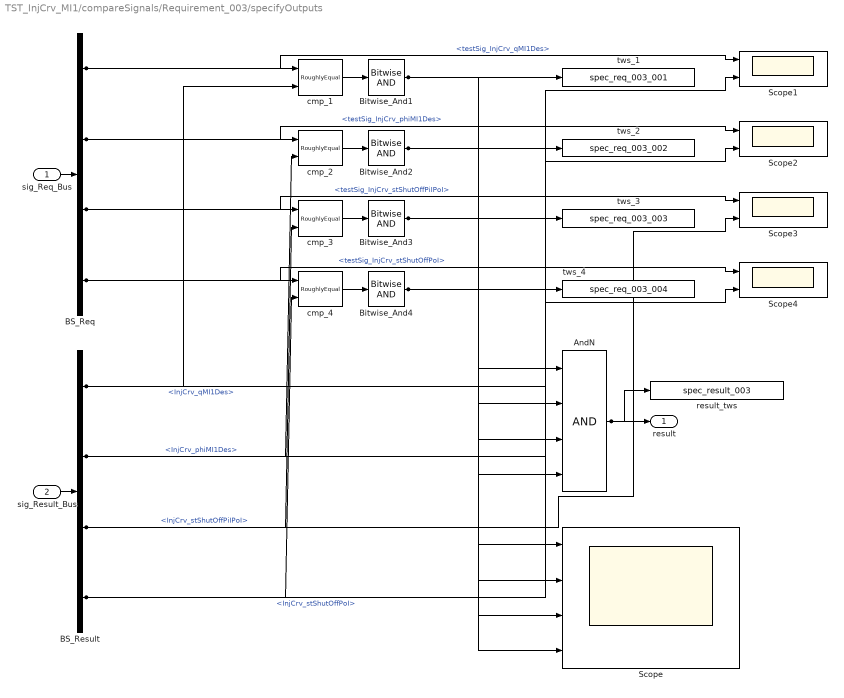
== system TST_InjCrv_MI1/compareSignals/Requirement_003/specifyOutputs ==
  sig_Req_Bus : Inport
  sig_Result_Bus : Inport  Port=2
  AndN : Logic  Inputs=4
  BS_Req : BusSelector  OutputSignals=testSig_InjCrv_qMI1Des,testSig_InjCrv_phiMI1Des,testSig_InjCrv_stShutOffPiIPoI,testSig_InjCrv_stShutOffPoI
  BS_Result : BusSelector  OutputSignals=InjCrv_qMI1Des,InjCrv_phiMI1Des,InjCrv_stShutOffPiIPoI,InjCrv_stShutOffPoI
  Bitwise_And{1..4} (4 alike) : simulink/Logic and Bit Operations/Bitwise Operator  logicop=AND  UseBitMask=off  BitMask=bin2dec('11011001')  BitMaskRealWorld=Stored Integer
  Scope : Scope  NumInputPorts=4
  Scope{1..4} (4 alike) : Scope  NumInputPorts=2
  cmp_{1..4} (4 alike) : UnitTest_Lib/RoughlyEqual  slope=0.1
  result_tws : ToWorkspace  VariableName=spec_result_003
  tws_1 : ToWorkspace  VariableName=spec_req_003_001
  tws_2 : ToWorkspace  VariableName=spec_req_003_002
  tws_3 : ToWorkspace  VariableName=spec_req_003_003
  tws_4 : ToWorkspace  VariableName=spec_req_003_004
  result : Outport
  wires:
  sig_Req_Bus/1 -> BS_Req/1
  sig_Result_Bus/1 -> BS_Result/1
  AndN/1 -> result/1, result_tws/1
  BS_Req/1 -> cmp_1/1, Scope1/1  "<testSig_InjCrv_qMI1Des>"
  BS_Result/1 -> cmp_1/2, Scope1/2  "<InjCrv_qMI1Des>"
  cmp_1/1 -> Bitwise_And1/1
  Bitwise_And1/1 -> tws_1/1, AndN/1, Scope/1
  BS_Req/2 -> cmp_2/1, Scope2/1  "<testSig_InjCrv_phiMI1Des>"
  BS_Result/2 -> cmp_2/2, Scope2/2  "<InjCrv_phiMI1Des>"
  cmp_2/1 -> Bitwise_And2/1
  Bitwise_And2/1 -> tws_2/1, AndN/2, Scope/2
  BS_Req/3 -> cmp_3/1, Scope3/1  "<testSig_InjCrv_stShutOffPiIPoI>"
  BS_Result/3 -> cmp_3/2, Scope3/2  "<InjCrv_stShutOffPiIPoI>"
  cmp_3/1 -> Bitwise_And3/1
  Bitwise_And3/1 -> tws_3/1, AndN/3, Scope/3
  BS_Req/4 -> cmp_4/1, Scope4/1  "<testSig_InjCrv_stShutOffPoI>"
  BS_Result/4 -> cmp_4/2, Scope4/2  "<InjCrv_stShutOffPoI>"
  cmp_4/1 -> Bitwise_And4/1
  Bitwise_And4/1 -> tws_4/1, AndN/4, Scope/4

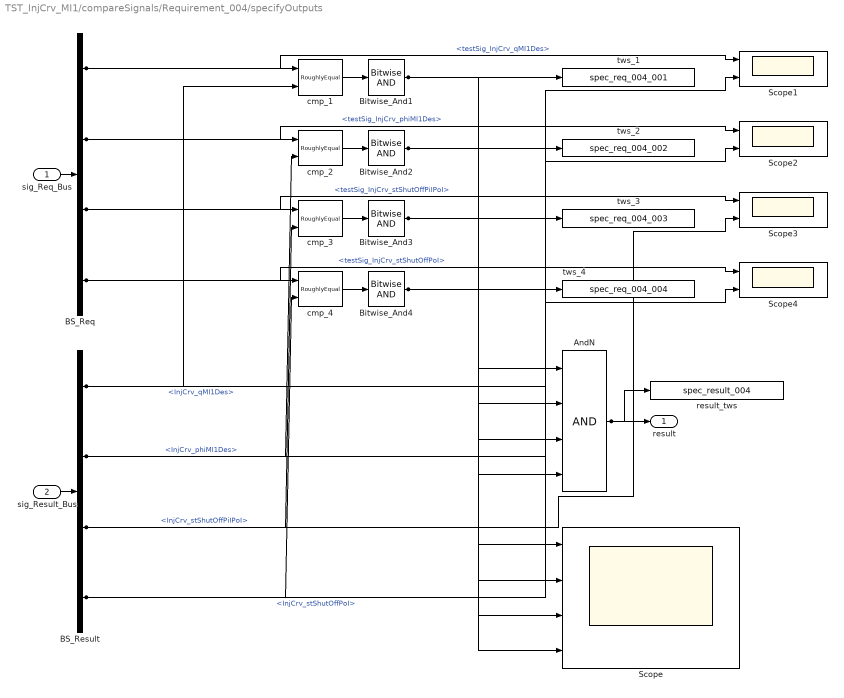
== system TST_InjCrv_MI1/compareSignals/Requirement_004/specifyOutputs ==
  sig_Req_Bus : Inport
  sig_Result_Bus : Inport  Port=2
  AndN : Logic  Inputs=4
  BS_Req : BusSelector  OutputSignals=testSig_InjCrv_qMI1Des,testSig_InjCrv_phiMI1Des,testSig_InjCrv_stShutOffPiIPoI,testSig_InjCrv_stShutOffPoI
  BS_Result : BusSelector  OutputSignals=InjCrv_qMI1Des,InjCrv_phiMI1Des,InjCrv_stShutOffPiIPoI,InjCrv_stShutOffPoI
  Bitwise_And{1..4} (4 alike) : simulink/Logic and Bit Operations/Bitwise Operator  logicop=AND  UseBitMask=off  BitMask=bin2dec('11011001')  BitMaskRealWorld=Stored Integer
  Scope : Scope  NumInputPorts=4
  Scope{1..4} (4 alike) : Scope  NumInputPorts=2
  cmp_{1..4} (4 alike) : UnitTest_Lib/RoughlyEqual  slope=0.1
  result_tws : ToWorkspace  VariableName=spec_result_004
  tws_1 : ToWorkspace  VariableName=spec_req_004_001
  tws_2 : ToWorkspace  VariableName=spec_req_004_002
  tws_3 : ToWorkspace  VariableName=spec_req_004_003
  tws_4 : ToWorkspace  VariableName=spec_req_004_004
  result : Outport
  wires:
  sig_Req_Bus/1 -> BS_Req/1
  sig_Result_Bus/1 -> BS_Result/1
  AndN/1 -> result/1, result_tws/1
  BS_Req/1 -> cmp_1/1, Scope1/1  "<testSig_InjCrv_qMI1Des>"
  BS_Result/1 -> cmp_1/2, Scope1/2  "<InjCrv_qMI1Des>"
  cmp_1/1 -> Bitwise_And1/1
  Bitwise_And1/1 -> tws_1/1, AndN/1, Scope/1
  BS_Req/2 -> cmp_2/1, Scope2/1  "<testSig_InjCrv_phiMI1Des>"
  BS_Result/2 -> cmp_2/2, Scope2/2  "<InjCrv_phiMI1Des>"
  cmp_2/1 -> Bitwise_And2/1
  Bitwise_And2/1 -> tws_2/1, AndN/2, Scope/2
  BS_Req/3 -> cmp_3/1, Scope3/1  "<testSig_InjCrv_stShutOffPiIPoI>"
  BS_Result/3 -> cmp_3/2, Scope3/2  "<InjCrv_stShutOffPiIPoI>"
  cmp_3/1 -> Bitwise_And3/1
  Bitwise_And3/1 -> tws_3/1, AndN/3, Scope/3
  BS_Req/4 -> cmp_4/1, Scope4/1  "<testSig_InjCrv_stShutOffPoI>"
  BS_Result/4 -> cmp_4/2, Scope4/2  "<InjCrv_stShutOffPoI>"
  cmp_4/1 -> Bitwise_And4/1
  Bitwise_And4/1 -> tws_4/1, AndN/4, Scope/4

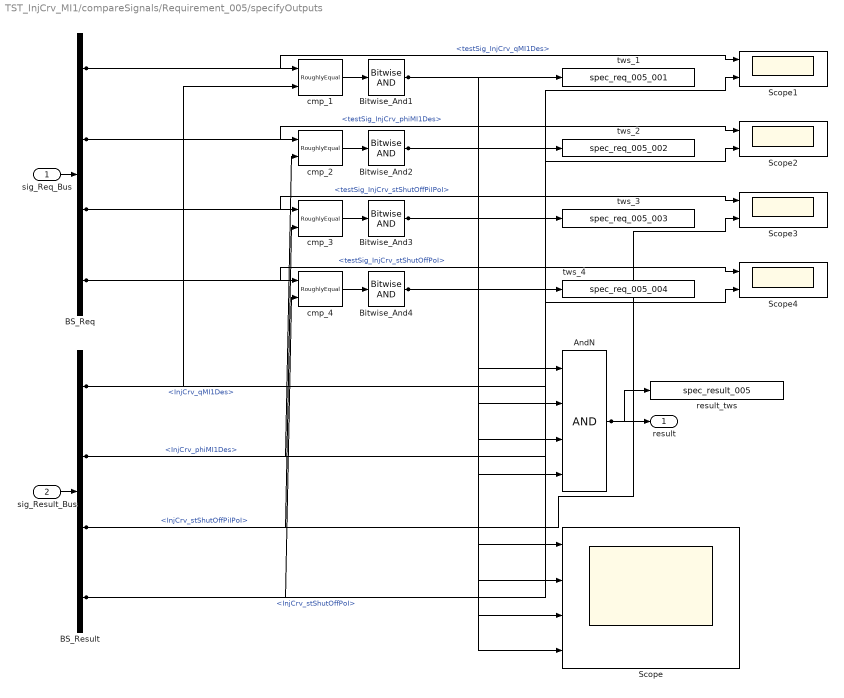
== system TST_InjCrv_MI1/compareSignals/Requirement_005/specifyOutputs ==
  sig_Req_Bus : Inport
  sig_Result_Bus : Inport  Port=2
  AndN : Logic  Inputs=4
  BS_Req : BusSelector  OutputSignals=testSig_InjCrv_qMI1Des,testSig_InjCrv_phiMI1Des,testSig_InjCrv_stShutOffPiIPoI,testSig_InjCrv_stShutOffPoI
  BS_Result : BusSelector  OutputSignals=InjCrv_qMI1Des,InjCrv_phiMI1Des,InjCrv_stShutOffPiIPoI,InjCrv_stShutOffPoI
  Bitwise_And{1..4} (4 alike) : simulink/Logic and Bit Operations/Bitwise Operator  logicop=AND  UseBitMask=off  BitMask=bin2dec('11011001')  BitMaskRealWorld=Stored Integer
  Scope : Scope  NumInputPorts=4
  Scope{1..4} (4 alike) : Scope  NumInputPorts=2
  cmp_{1..4} (4 alike) : UnitTest_Lib/RoughlyEqual  slope=0.1
  result_tws : ToWorkspace  VariableName=spec_result_005
  tws_1 : ToWorkspace  VariableName=spec_req_005_001
  tws_2 : ToWorkspace  VariableName=spec_req_005_002
  tws_3 : ToWorkspace  VariableName=spec_req_005_003
  tws_4 : ToWorkspace  VariableName=spec_req_005_004
  result : Outport
  wires:
  sig_Req_Bus/1 -> BS_Req/1
  sig_Result_Bus/1 -> BS_Result/1
  AndN/1 -> result/1, result_tws/1
  BS_Req/1 -> cmp_1/1, Scope1/1  "<testSig_InjCrv_qMI1Des>"
  BS_Result/1 -> cmp_1/2, Scope1/2  "<InjCrv_qMI1Des>"
  cmp_1/1 -> Bitwise_And1/1
  Bitwise_And1/1 -> tws_1/1, AndN/1, Scope/1
  BS_Req/2 -> cmp_2/1, Scope2/1  "<testSig_InjCrv_phiMI1Des>"
  BS_Result/2 -> cmp_2/2, Scope2/2  "<InjCrv_phiMI1Des>"
  cmp_2/1 -> Bitwise_And2/1
  Bitwise_And2/1 -> tws_2/1, AndN/2, Scope/2
  BS_Req/3 -> cmp_3/1, Scope3/1  "<testSig_InjCrv_stShutOffPiIPoI>"
  BS_Result/3 -> cmp_3/2, Scope3/2  "<InjCrv_stShutOffPiIPoI>"
  cmp_3/1 -> Bitwise_And3/1
  Bitwise_And3/1 -> tws_3/1, AndN/3, Scope/3
  BS_Req/4 -> cmp_4/1, Scope4/1  "<testSig_InjCrv_stShutOffPoI>"
  BS_Result/4 -> cmp_4/2, Scope4/2  "<InjCrv_stShutOffPoI>"
  cmp_4/1 -> Bitwise_And4/1
  Bitwise_And4/1 -> tws_4/1, AndN/4, Scope/4
